simulink model "buck_converter"  (R2021b)
settings: Solver=VariableStepAuto  StartTime=0.0  StopTime=0.2  FixedStep=1e-6  MaxStep=1e-5  RelTol=1e-3
libraries: spsSeriesRLCBranchLib x3, spsMeanLib x2, spsDiodeLib x1, spsIGBTDiodeLib x1, spsCurrentMeasurementLib x1, spsDCVoltageSourceLib x1, spsVoltageMeasurementLib x1, spspowerguiLib x1
settings Model: Creator=Vishal  LastModifiedBy=Vishal

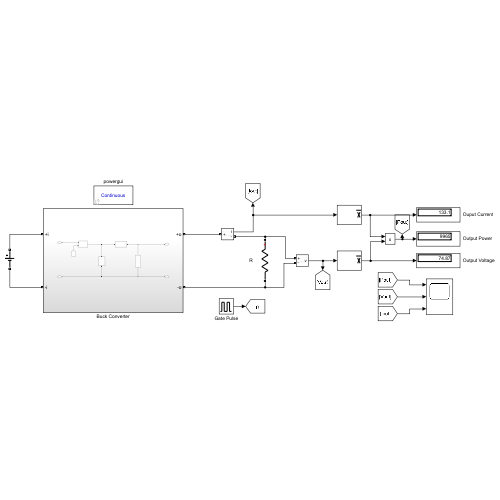
[thumbnail: Simulink's stored preview of the top-level diagram]
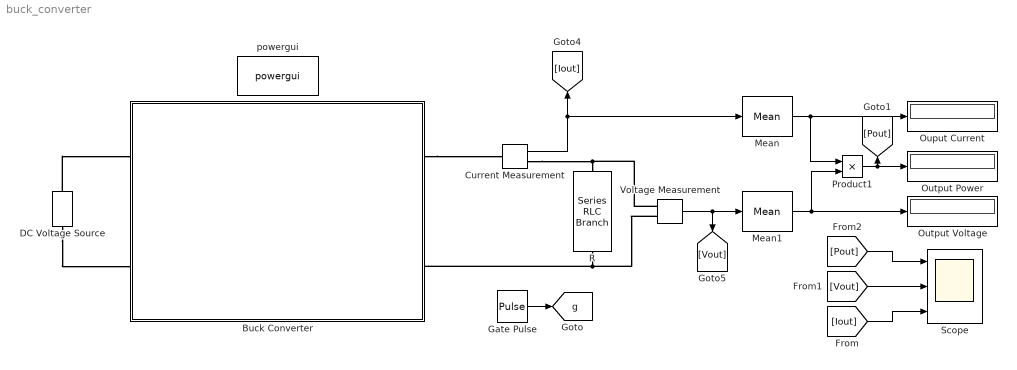
== system buck_converter ==
  Buck Converter : Subsystem
  Current Measurement : spsCurrentMeasurementLib/Current Measurement  PhasorSimulation=off  OutputType=Complex  PSBequivalent=0
  DC Voltage Source : spsDCVoltageSourceLib/DC Voltage Source  Amplitude=150  Measurements=None
  Gate Pulse : DiscretePulseGenerator  PulseType=Time based  Period=1/50000  PulseWidth=50
  Mean : spsMeanLib/Mean  Freq=50000  Vinit=0  Ts=0
  Mean1 : spsMeanLib/Mean  Freq=50000  Vinit=0  Ts=0
  Ouput Current : Display
  Output Power : Display
  Output Voltage : Display
  Product1 : Product
  R : spsSeriesRLCBranchLib/Series RLC Branch  LConnTagsString=__new0  RConnTagsString=__new0  BranchType=R  Resistance=0.5625  Inductance=1e-3  SetiL0=off  InitialCurrent=0  Capacitance=1e-6  Setx0=off  InitialVoltage=0  Measurements=None
  Scope : Scope  NumInputPorts=3
  Voltage Measurement : spsVoltageMeasurementLib/Voltage Measurement  PhasorSimulation=off  OutputType=Complex  PSBequivalent=0
  powergui : spspowerguiLib/powergui  Priority=1  SimulationMode=Continuous  SampleTime=50e-6  frequency=60  Iterations=50  frequencyindice=0  Pbase=100e6  ErrMax=1e-4  UnitsV=kV  UnitsW=MW  buscounter=0  FunctionMessages=off  echomessages=off  EnableUseOfTLC=off  CurrentSourceSwitches=off  DisableSnubberDevices=off  DisableRonSwitches=off  DisableVfSwitches=off  DisplayEquations=off  AutomaticDiscreteSolvers=off  SolverType=Tustin/Backward Euler (TBE)  Interpol=off  ExternalGateDelay=off  methode=off  Ts=100  x0status=blocks  SPID=on  SwTol=0  HookPort=off  NonlinearTolerance=1e-4  nMaxIteration=100  ContinueOnMaxIteration=off  RestoreLinks=warning  ResistiveCurrentMeasurement=off  Frange=[0:2:500]  Ylog=off  Xlog=on  ShowGrid=off  save=off  variable=ZData  structure=0  ZoomFFT=off  StartTime=0.0  cycles=1  DisplayStyle=1  fundamental=60  FreqAxis=off  MaxFrequency=1000  frequencyindicesteady=1  RmsSteady=1  display=off
  tag scope: g=global
  wires:
  Product1/1 -> Output Power/1, [Pout]
  Current Measurement/1 -> [Iout], Mean/1
  Mean/1 -> Product1/1, Ouput Current/1
  Mean1/1 -> Output Voltage/1, Product1/2
  Voltage Measurement/1 -> Mean1/1, [Vout]
  [Vout] -> Scope/2
  [Iout] -> Scope/3
  [Pout] -> Scope/1
  Gate Pulse/1 -> [g]
  connections:
  Voltage Measurement/LConn1 -- R/LConn1 -- Current Measurement/RConn1
  R/RConn1 -- Voltage Measurement/LConn2 -- Buck Converter/RConn2
  DC Voltage Source/RConn1 -- Buck Converter/LConn1
  DC Voltage Source/LConn1 -- Buck Converter/LConn2
  Buck Converter/RConn1 -- Current Measurement/LConn1

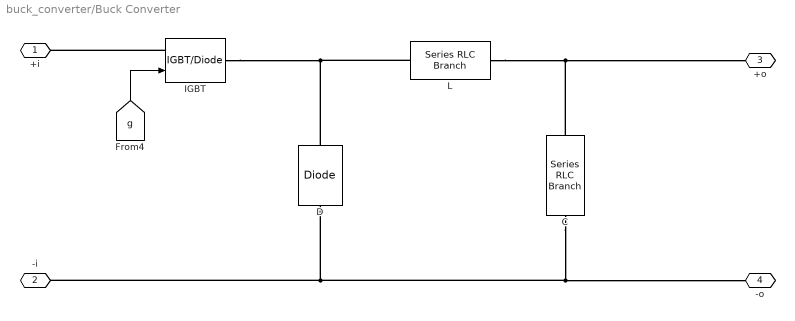
== system buck_converter/Buck Converter ==
  C : spsSeriesRLCBranchLib/Series RLC Branch  LConnTagsString=__new0  RConnTagsString=__new0  BranchType=C  Resistance=1e-4  Inductance=1e-3  SetiL0=off  InitialCurrent=0  Capacitance=2.2222e-05  Setx0=off  InitialVoltage=0  Measurements=None
  D : spsDiodeLib/Diode  Ron=0.001  Lon=0  Vf=0  IC=0  UseSnubber=0  Rs=500  Cs=250e-9  Measurements=off
  IGBT : spsIGBTDiodeLib/IGBT//Diode  Ron=1e-3  Rs=1e5  Cs=inf  Measurements=off
  L : spsSeriesRLCBranchLib/Series RLC Branch  LConnTagsString=__new0  RConnTagsString=__new0  BranchType=L  Resistance=0.1  Inductance=1.1250e-04  SetiL0=off  InitialCurrent=0  Capacitance=1e-6  Setx0=off  InitialVoltage=0  Measurements=None
  +i : PMIOPort  Side=Left
  -i : PMIOPort  Port=2  Side=Left
  +o : PMIOPort  Port=3  Side=Right
  -o : PMIOPort  Port=4  Side=Right
  wires:
  [g] -> IGBT/1
  connections:
  IGBT/LConn1 -- +i/RConn1
  C/LConn1 -- L/RConn1 -- +o/RConn1
  IGBT/RConn1 -- D/RConn1 -- L/LConn1
  C/RConn1 -- -i/RConn1 -- D/LConn1 -- -o/RConn1
